simulink model "Filter_Bank_Model"  (R2020b)
settings: Solver=FixedStepDiscrete  StartTime=0.0  StopTime=100  RelTol=1e-3
undefined symbols (not defined in the file or in its folder): fdesignblkfcn, gcbh, magnitude
libraries: dspfdesign x2, commrandsrc3 x1, commrflib2 x1, commdigbbndpm3 x1, commfilt2 x1, dspsrcs4 x1
settings Model: Creator=J72373  LastModifiedBy=harme
settings SolverCC: AutoInsertRateTranBlk=on
settings DataIOCC: SaveOutput=off  SignalLogging=off  SaveTime=off

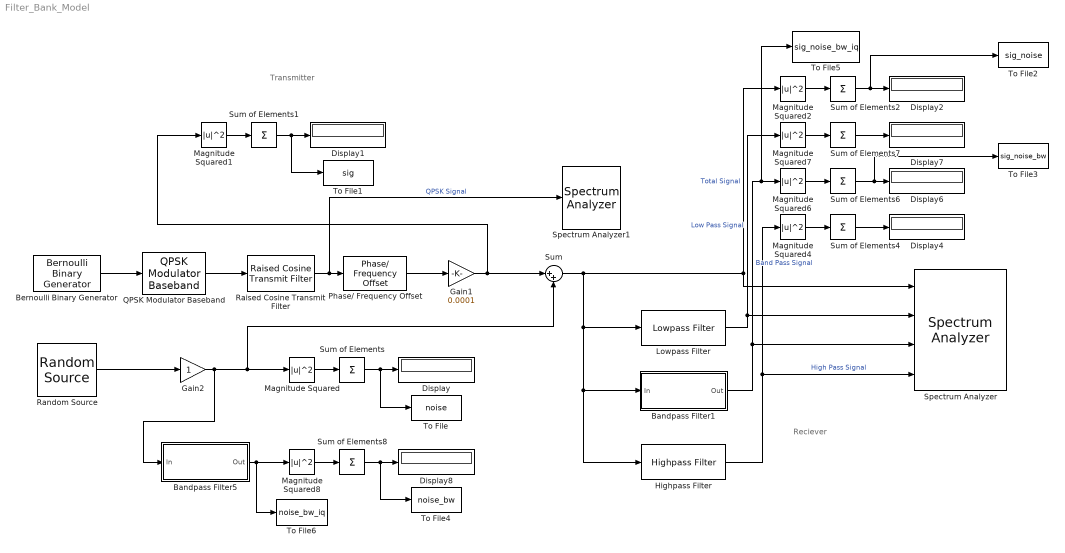
== system Filter_Bank_Model ==
  note: Transmitter
  note: Reciever
  Bandpass Filter1 : Subsystem  DialogController=fdesignblkfcn  InitFcn=fdesignblkfcn(gcbh, {'InitFcn'});  mask(Bandpass Filter){}
      mask help: Design a bandpass filter
      settings: CopyFcn=fdesignblkfcn(gcbh, {'CopyFcn'});
      mask Help: helpview(mapfilelocation('dsp'), 'dspbandpassfilter');
      mask Display: disp('Bandpass');
  Bandpass Filter5 : Subsystem  DialogController=fdesignblkfcn  InitFcn=fdesignblkfcn(gcbh, {'InitFcn'});  mask(Bandpass Filter){}
      mask help: Design a bandpass filter
      settings: CopyFcn=fdesignblkfcn(gcbh, {'CopyFcn'});
      mask Help: helpview(mapfilelocation('dsp'), 'dspbandpassfilter');
      mask Display: disp('Bandpass');
  Bernoulli Binary Generator : commrandsrc3/Bernoulli Binary Generator  ProbabilityOfZero=0.5  SeedSource=Auto  Seed=0  SampleTime=-1  SamplesPerFrame=40  OutputDataType=double  SimulateUsing=Interpreted execution
  Display{,1..2,4,6..8} (7 alike) : Display
  Gain1 : Gain  Gain=0.0001
  Gain2 : Gain
  Highpass Filter : dspfdesign/Highpass Filter  FilterType=FIR  DesignForMinimumOrder=on  FilterOrder=50  StopbandFrequency=14e3  PassbandFrequency=16e3  StopbandAttenuation=70  PassbandRipple=0.1  InheritSampleRate=off  SampleRate=44100  SimulateUsing=Interpreted execution  roundingMode=Floor  coeffsDataTypeStr=fixdt(1,16)
  Lowpass Filter : dspfdesign/Lowpass Filter  FilterType=FIR  DesignForMinimumOrder=on  FilterOrder=50  PassbandFrequency=5e3  StopbandFrequency=7e3  PassbandRipple=0.1  StopbandAttenuation=70  InheritSampleRate=off  SampleRate=44100  SimulateUsing=Interpreted execution  roundingMode=Floor  coeffsDataTypeStr=fixdt(1,16)
  Magnitude Squared{,1..2,4,6..8} (7 alike) : Math  Operator=magnitude^2  SaturateOnIntegerOverflow=on
  Phase/ Frequency Offset : commrflib2/Phase// Frequency Offset  phaseOffset=0  freqPort=off  freqOffset=11000
  QPSK Modulator Baseband : commdigbbndpm3/QPSK Modulator Baseband  InType=Bit  Enc=Gray  Ph=pi/4  outDtype=double  outWordLen=16  outUDDataType=sfix(16)  outFracLenMode=Best precision  outFracLen=15  outDataTypeStr=double  outLastDataTypeStr=double
  Raised Cosine Transmit Filter : commfilt2/Raised Cosine Transmit Filter  filtType=Square root  R=0.2  filtSpan=32  N=10  filterGain=1  InputProcessing=Columns as channels (frame based)  RateOptions=Enforce single-rate processing  framing=Mute  checkCoeff=off  variableName=rcTxFilt  checkGain=Normalized  sampMode=Mute  saveAsFlag=0  currentFiltSpan=32  D=(32)/2  launchFVT=on  roundingMode=Floor  overflowMode=off  coeffDataTypeStr=Inherit: Same word length as input  coeffMin=[]  coeffMax=[]  coeffLastDataTypeStr=Inherit: Same word length as input  outputDataTypeStr=Inherit: Same as accumulator  outputMin=[]  outputMax=[]  outputLastDataTypeStr=Inherit: Same as accumulator
  Random Source : dspsrcs4/Random Source  SrcType=Gaussian  NormMethod=Ziggurat  CltLength=12  MinVal=0  MaxVal=1  MeanVal=0  VarVal=0.05  RepMode=Specify seed  rawSeed=1234567  IsInherit=off  SampMode=Discrete  SampTime=1/44100  SampFrame=200  DataType=Double  OutComplex=Complex  OutputFrames=off
  Spectrum Analyzer : SpectrumAnalyzer  NumInputPorts=4
  Spectrum Analyzer1 : SpectrumAnalyzer
  Sum : Sum  Inputs=|++
  Sum of Elements{,1..2,4,6..8} (7 alike) : Sum  Inputs=+
  To File : ToFile  Filename=noise  SaveFormat=Timeseries
  To File1 : ToFile  Filename=sig  SaveFormat=Timeseries
  To File2 : ToFile  Filename=sig_noise  SaveFormat=Timeseries
  To File3 : ToFile  Filename=sig_noise_bw  SaveFormat=Timeseries
  To File4 : ToFile  Filename=noise_bw  SaveFormat=Timeseries
  To File5 : ToFile  Filename=sig_noise_bw_iq  SaveFormat=Timeseries
  To File6 : ToFile  Filename=noise_bw_iq  SaveFormat=Timeseries
  wires:
  Bernoulli Binary Generator/1 -> QPSK Modulator Baseband/1
  Raised Cosine Transmit Filter/1 -> Spectrum Analyzer1/1, Phase/ Frequency Offset/1  "QPSK Signal"
  Phase/ Frequency Offset/1 -> Gain1/1
  QPSK Modulator Baseband/1 -> Raised Cosine Transmit Filter/1
  Magnitude Squared/1 -> Sum of Elements/1
  Sum of Elements/1 -> To File/1, Display/1
  Gain1/1 -> Magnitude Squared1/1, Sum/1
  Sum/1 -> Magnitude Squared2/1, Spectrum Analyzer/1, Lowpass Filter/1, Highpass Filter/1, Bandpass Filter1/1(In)  "Total Signal"
  Sum of Elements1/1 -> To File1/1, Display1/1
  Magnitude Squared1/1 -> Sum of Elements1/1
  Magnitude Squared2/1 -> Sum of Elements2/1
  Sum of Elements2/1 -> To File2/1, Display2/1
  Random Source/1 -> Gain2/1
  Gain2/1 -> Bandpass Filter5/1(In), Sum/2, Magnitude Squared/1
  Lowpass Filter/1 -> Magnitude Squared7/1, Spectrum Analyzer/2  "Low Pass Signal"
  Bandpass Filter1/1(Out) -> To File5/1, Magnitude Squared6/1, Spectrum Analyzer/3  "Band Pass Signal"
  Highpass Filter/1 -> Spectrum Analyzer/4, Magnitude Squared4/1  "High Pass Signal"
  Sum of Elements4/1 -> Display4/1
  Magnitude Squared4/1 -> Sum of Elements4/1
  Sum of Elements6/1 -> To File3/1, Display6/1
  Magnitude Squared6/1 -> Sum of Elements6/1
  Sum of Elements7/1 -> Display7/1
  Magnitude Squared7/1 -> Sum of Elements7/1
  Sum of Elements8/1 -> To File4/1, Display8/1
  Magnitude Squared8/1 -> Sum of Elements8/1
  Bandpass Filter5/1(Out) -> To File6/1, Magnitude Squared8/1

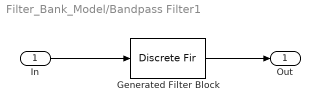
== system Filter_Bank_Model/Bandpass Filter1 ==
  In : Inport
  Generated Filter Block : DiscreteFir  Tag=BlockMethodSubSystem  Coefficients=[-0.00121889259374306043 -4.6471804164866279e-08 0.0022568060688219157 1.71088361680865877e-07 0.00277263523316290464 -3.91787000503089673e-07 -0.0194126295457396937 5.96679699808125005e-07 0.0393950026121096392 -6.5164419275998585e-07 -0.0344159794027284888 4.7046709147951619e-07 -0.0257306182897297508 -1.75073104912854821e-07 0.138632970079688084 -4.06676534540085174e-08 -0.253908540757038725 4.57124845899172159e-08 0.30300878215917032 4.57124845899172159e-08 -0.253908540757038725 -4.06676534540085174e-08 0.138632970079688084 -1.75073104912854821e-07 -0.0257306182897297508 4.7046709147951619e-07 -0.0344159794027284888 -6.5164419275998585e-07 0.0393950026121096392 5.96679699808125005e-07 -0.0194126295457396937 -3.91787000503089673e-07 0.00277263523316290464 1.71088361680865877e-07 0.0022568060688219157 -4.6471804164866279e-08 -0.00121889259374306043]  InputProcessing=Columns as channels (frame based)
  Out : Outport  VectorParamsAs1DForOutWhenUnconnected=off
  wires:
  In/1 -> Generated Filter Block/1
  Generated Filter Block/1 -> Out/1

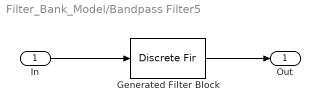
== system Filter_Bank_Model/Bandpass Filter5 ==
  In : Inport
  Generated Filter Block : DiscreteFir  Tag=BlockMethodSubSystem  Coefficients=[0.00732042010249847608 0.0106282918763365309 -0.00704818145835509492 -0.0139774864976023126 0.00139251813232264278 0.00103573235549302947 -0.0032720074229586559 0.00719192846207008032 0.00376555578256326622 0.00164698563023850625 0.0100490589250385037 0.00319517982739197376 0.00375186900268913246 0.0102804221955299854 0.000530639608501540564 0.00500797317880307107 0.00836056668232693263 -0.00276387666336760755 0.00597680195448394534 0.00460848835913731884 -0.00592991475429197491 0.00666059580252770841 -0.00108390978155830471 -0.00822294616576458269 0.00637879124089539128 -0.0085859166125103123 -0.00937442062776747478 0.00426849299810129999 -0.0174386043721060681 -0.00900965741455647673 -0.000604203193372156275 -0.0266925927525068427 -0.00711827439460679164 -0.00889853500440642223 -0.0348941431836110594 -0.00383458192104142856 -0.0211495280897720378 -0.040146200620220937 0.000392173673884891358 -0.0378015418392869326 -0.0400552045944938678 0.00488700111954579273 -0.0601639450933004541 -0.0305707332433210396 0.00885913220731158503 -0.0942290304307732141 0.00106110010169847163 0.0115964876108286923 -0.189327473672283919 0.214201226591654165 0.679242366448524759 0.214201226591654165 -0.189327473672283919 0.0115964876108286923 0.00106110010169847163 -0.0942290304307732141 0.00885913220731158503 -0.0305707332433210396 -0.0601639450933004541 0.00488700111954579273 -0.0400552045944938678 -0.0378015418392869326 0.000392173673884891358 -0.040146200620220937 -0.0211495280897720378 -0.00383458192104142856 -0.0348941431836110594 -0.00889853500440642223 -0.00711827439460679164 -0.0266925927525068427 -0.000604203193372156275 -0.00900965741455647673 -0.0174386043721060681 0.00426849299810129999 -0.00937442062776747478 -0.0085859166125103123 0.00637879124089539128 -0.00822294616576458269 -0.00108390978155830471 0.00666059580252770841 -0.00592991475429197491 0.00460848835913731884 0.00597680195448394534 -0.00276387666336760755 0.00836056668232693263 0.00500797317880307107 0.000530639608501540564 0.0102804221955299854 0.00375186900268913246 0.00319517982739197376 0.0100490589250385037 0.00164698563023850625 0.00376555578256326622 0.00719192846207008032 -0.0032720074229586559 0.00103573235549302947 0.00139251813232264278 -0.0139774864976023126 -0.00704818145835509492 0.0106282918763365309 0.00732042010249847608]  InputProcessing=Columns as channels (frame based)
  Out : Outport  VectorParamsAs1DForOutWhenUnconnected=off
  wires:
  In/1 -> Generated Filter Block/1
  Generated Filter Block/1 -> Out/1
